simulink model "prova"  (R2018b)
settings: Solver=ode4  StartTime=0.0  StopTime=inf  FixedStep=T  RelTol=1e-3
values from neighbouring files (symbols this model uses):
  T = 0.5    [MPC_kin_N=6arc traj.mat]    (also in MPC_kin_N=7complex traj_ultimo.mat = 0.2; MPC_kin_Param_N=10 traj_retta.mat = 0.4; MPC_kin_Param_N=10 traj_ultimo.mat = 0.4; Traj_Prova.m = 0.2)
undefined symbols (not defined in the file or in its folder): Angular, Linear
libraries: robotlib x3, sharedtransform x1, simulink x1
settings Model: EnablePacing=on  Creator=francesco  LastModifiedBy=francesco

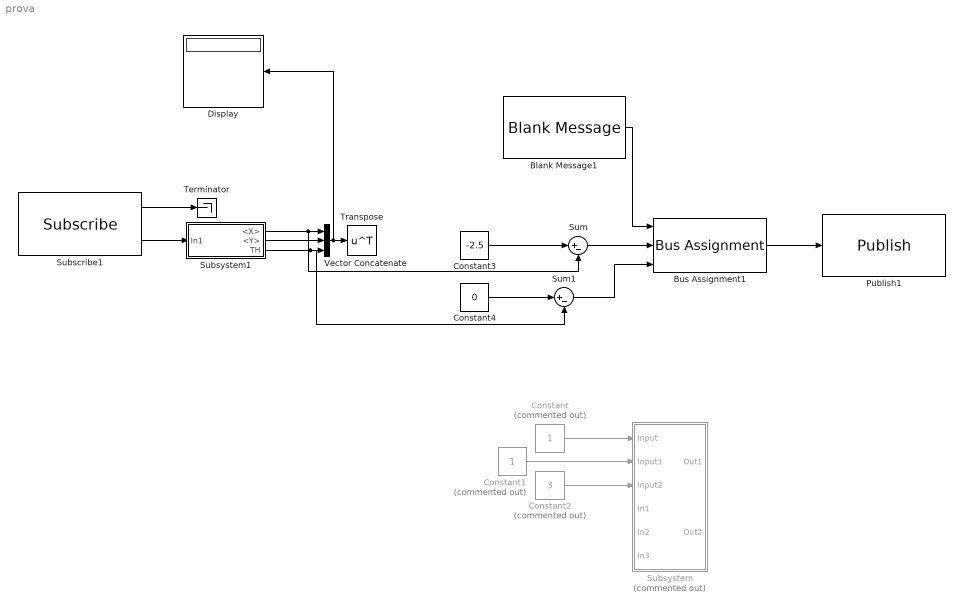
== system prova ==
  Blank Message1 : robotlib/Blank Message  messageClass=Message  entityType=geometry_msgs/Twist  messageType=geometry_msgs/Twist  SampleTime=T
      settings: SourceProductBaseCode=RO
  Bus Assignment1 : BusAssignment  AssignedSignals=Linear.X,Angular.Z
  Constant : Constant  Commented=on
  Constant1 : Constant  Commented=on
  Constant2 : Constant  Commented=on  Value=3
  Constant3 : Constant  Value=-2.5
  Constant4 : Constant  Value=0
  Display : Display
  Publish1 : robotlib/Publish  topicSource=Select from ROS network  topic=/husky_velocity_controller/cmd_vel  messageType=geometry_msgs/Twist  messageQueueLength=1
      settings: SourceProductBaseCode=RO
  Subscribe1 : robotlib/Subscribe  topicSource=Select from ROS network  topic=/odometry/filtered  messageType=nav_msgs/Odometry  sampleTime=T  messageQueueLength=1
      settings: SourceProductBaseCode=RO
  Subsystem : Subsystem  Commented=on
  Subsystem1 : Subsystem
  Sum : Sum  Inputs=|+-
  Sum1 : Sum  Inputs=|+-
  Terminator : Terminator
  Transpose : Math  Operator=transpose  SaturateOnIntegerOverflow=on
  Vector Concatenate : Concatenate  NumInputs=3
  wires:
  Blank Message1/1 -> Bus Assignment1/1
  Bus Assignment1/1 -> Publish1/1
  Subsystem1/1(<X>) -> Sum/2, Vector Concatenate/1
  Subsystem1/2(<Y>) -> Vector Concatenate/2
  Subsystem1/3(TH) -> Sum1/2, Vector Concatenate/3
  Subscribe1/1 -> Terminator/1
  Vector Concatenate/1 -> Display/1, Transpose/1
  Subscribe1/2 -> Subsystem1/1(In1)
  Constant2/1 -> Subsystem/3(Input2)
  Constant1/1 -> Subsystem/2(Input1)
  Constant/1 -> Subsystem/1(Input)
  Constant3/1 -> Sum/1
  Constant4/1 -> Sum1/1
  Sum/1 -> Bus Assignment1/2
  Sum1/1 -> Bus Assignment1/3

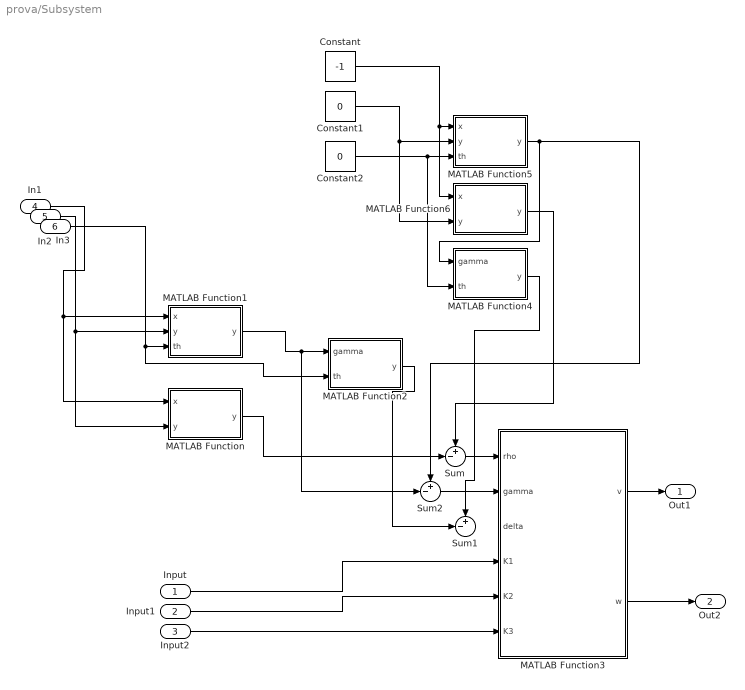
== system prova/Subsystem ==
  Input : Inport
  Input1 : Inport  Port=2
  Input2 : Inport  Port=3
  In1 : Inport  Port=4
  In2 : Inport  Port=5
  In3 : Inport  Port=6
  Constant : Constant  Value=-1
  Constant1 : Constant  Value=0
  Constant2 : Constant  Value=0
  MATLAB Function : MATLAB Function  TreatAsAtomicUnit=on
  MATLAB Function1 : MATLAB Function  TreatAsAtomicUnit=on
  MATLAB Function2 : MATLAB Function  TreatAsAtomicUnit=on
  MATLAB Function3 : MATLAB Function  TreatAsAtomicUnit=on
  MATLAB Function4 : MATLAB Function  TreatAsAtomicUnit=on
  MATLAB Function5 : MATLAB Function  TreatAsAtomicUnit=on
  MATLAB Function6 : MATLAB Function  TreatAsAtomicUnit=on
  Sum : Sum  Inputs=+-|
  Sum1 : Sum  Inputs=+-|
  Sum2 : Sum  Inputs=+-|
  Out1 : Outport
  Out2 : Outport  Port=2
  wires:
  In2/1 -> MATLAB Function/2("y "), MATLAB Function1/2("y ")
  MATLAB Function1/1(y) -> Sum2/2, MATLAB Function2/1(gamma)
  MATLAB Function3/2(w) -> Out2/1
  In3/1 -> MATLAB Function2/2(th), MATLAB Function1/3(th)
  Input2/1 -> MATLAB Function3/6(K3)
  MATLAB Function3/1(v) -> Out1/1
  Input/1 -> MATLAB Function3/4(K1)
  In1/1 -> MATLAB Function/1(x), MATLAB Function1/1(x)
  Input1/1 -> MATLAB Function3/5(K2)
  Constant/1 -> MATLAB Function6/1(x), MATLAB Function5/1(x)
  Constant1/1 -> MATLAB Function6/2("y "), MATLAB Function5/2("y ")
  Constant2/1 -> MATLAB Function4/2(th), MATLAB Function5/3(th)
  MATLAB Function5/1(y) -> Sum2/1, MATLAB Function4/1(gamma)
  Sum/1 -> MATLAB Function3/1(rho)
  Sum2/1 -> MATLAB Function3/2(gamma)
  MATLAB Function/1(y) -> Sum/2
  MATLAB Function6/1(y) -> Sum/1
  MATLAB Function2/1(y) -> Sum1/2
  MATLAB Function4/1(y) -> Sum1/1

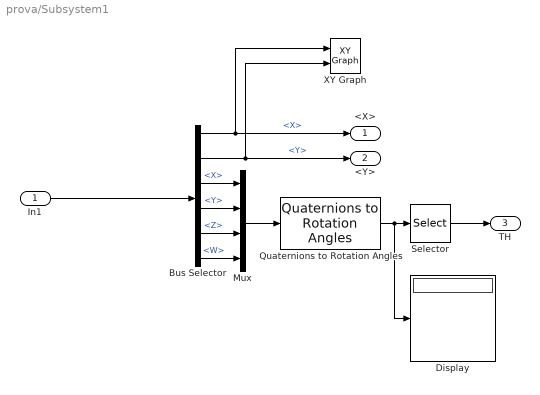
== system prova/Subsystem1 ==
  In1 : Inport
  Bus Selector : BusSelector  OutputSignals=Pose.Pose.Position.X,Pose.Pose.Position.Y,Pose.Pose.Orientation.X,Pose.Pose.Orientation.Y,Pose.Pose.Orientation.Z,Pose.Pose.Orientation.W
  Display : Display
  Mux : Mux
  Quaternions to Rotation Angles : sharedtransform/Quaternions to Rotation Angles  rotationOrder=ZYX  aMode=aMode
      settings: SourceProductBaseCode=AE
  Selector : Selector  InputPortWidth=3  IndexOptions=Index vector (dialog)  Indices=3  OutputSizes=1
  XY Graph : simulink/Sinks/XY Graph  xmin=-1  xmax=8  ymin=-1  ymax=8  st=-1
  <X> : Outport
  <Y> : Outport  Port=2
  TH : Outport  Port=3
  wires:
  Bus Selector/1 -> XY Graph/1, <X>/1  "<X>"
  In1/1 -> Bus Selector/1
  Bus Selector/2 -> XY Graph/2, <Y>/1  "<Y>"
  Bus Selector/6 -> Mux/4  "<W>"
  Bus Selector/5 -> Mux/3  "<Z>"
  Bus Selector/4 -> Mux/2  "<Y>"
  Bus Selector/3 -> Mux/1  "<X>"
  Mux/1 -> Quaternions to Rotation Angles/1
  Quaternions to Rotation Angles/1 -> Display/1, Selector/1
  Selector/1 -> TH/1

== matlab function prova/Subsystem/MATLAB Function1 ==
  data: x input; y output; y input; th input
function y = gamma(x,y,th)

y=atan2(y,x)-th+pi;

== matlab function prova/Subsystem/MATLAB Function ==
  data: x input; y output; y input
function y = rho(x,y)

y=sqrt(x^2+y^2);

== matlab function prova/Subsystem/MATLAB Function2 ==
  data: gamma input; y output; th input
function y = delta(gamma,th)

y = gamma+th;

== matlab function prova/Subsystem/MATLAB Function3 ==
  data: rho input; v output; gamma input; delta input; K1 input; K2 input; K3 input; w output
function [v,w] = fcn(rho,gamma,delta,K1,K2,K3)

v=K1*rho*cos(gamma);
w=K2*gamma+K1*((sin(gamma)*cos(gamma))/gamma)*(gamma+K3*delta)

== matlab function prova/Subsystem/MATLAB Function4 ==
  data: gamma input; y output; th input
function y = delta(gamma,th)

y = gamma+th;

== matlab function prova/Subsystem/MATLAB Function5 ==
  data: x input; y output; y input; th input
function y = gamma(x,y,th)

y=atan2(y,x)-th+pi;

== matlab function prova/Subsystem/MATLAB Function6 ==
  data: x input; y output; y input
function y = rho(x,y)

y=sqrt(x^2+y^2);
